simulink model "PassVeh7DOF"  (R2024b)
settings: Solver=ode14x  StartTime=0.0  StopTime=30  FixedStep=0.001  RelTol=1e-1
model workspace (MAT data in the model file):
  A_mu = 10
  B_reff = 8.386
  CONVERTER_DATA = [0 0.1 0.2 0.3 0.4 0.5 0.6 0.7 0.8 0.81 0.82 0.83 ... (63 elements, 21x3)]
  Cps = 2
  Cz = 7766.25
  DOWN_TABLE = [0 0 0 0 0 0 5 5 7.5 7.5 15 15 ... (30 elements, 6x5)]
  DOWN_TH_BP = [0 5 40 50 90 100]
  D_reff = 0.25826
  EMAP = [-40 215 245 264 264 267 267 267 267 267 -44 117 ... (110 elements, 10x11)]
  F0z = [6086.4 4324.8]
  F_reff = 0.07394
  F_zmax = 10000
  F_zmin = 100
  F_zo = 4000
  Kz = 48000
  MF : object (value not decoded)
  NCyl = 6
  NE_VEC = [800 1200 1600 2000 2400 2800 3200 3600 4000 4400 4800]
  Pstd = 101325
  R_eff = 0.298
  Rair = 287
  SUS : object (value not decoded)
  TH_VEC = [0; 20; 30; 40; 50; 60; 70; 80; 90; 100]
  TWAITdn = 1.25
  TWAITup = 0.1
  Tin = [1 2 3 4 5 6 7 8 9 10 2 2 ... (20 elements, 10x2)]
  Tstd = 293.15
  UP_TABLE = [7.5 7.5 15 25 40 40 25 25 35 45 70 80 ... (30 elements, 6x5)]
  UP_TH_BP = [0 25 35 50 90 100]
  VEH : object (value not decoded)
  V_o = 16.7
  V_xlow = 1
  Vd = 0.00346
  WH : object (value not decoded)
  a = 1.515
  alpha_max = 1.5
  alpha_min = -1.5
  b = 1.504
  c_zo = 209651
  epsilon = 0.1
  f_air = [0 0 0 0 0 0 0 0 0 0 0 0 ... (256 elements, 16x16)]
  f_co = [0 0 0 0 0 0 0 0 0 0 0 0 ... (256 elements, 16x16)]
  f_co2 = [0 0 0 0 0 0 0 0 0 0 0 0 ... (256 elements, 16x16)]
  f_eff = [352.135682859 352.135682859 320.724378192 303.655312657 295.930136708 291.240087194 291.240271258 291.240312459 291.240275452 291.240198499 291.240100781 291.240018769 ... (256 elements, 16x16)]
  f_fuel = [0 0 0 0 0 0 0 0 0 0 0 0 ... (256 elements, 16x16)]
  f_hc = [0 0 0 0 0 0 0 0 0 0 0 0 ... (256 elements, 16x16)]
  f_nox = [0 0 0 0 0 0 0 0 0 0 0 0 ... (256 elements, 16x16)]
  f_pm = [0 0 0 0 0 0 0 0 0 0 0 0 ... (256 elements, 16x16)]
  f_susp_axl_bp = [1 2]
  f_susp_dz_bp = [-4 -0.14 -0.13 -0.12 -0.11 -0.1 -0.09 -0.08 -0.07 -0.06 -0.05 -0.04 ... (31 elements, 1x31)]
  f_susp_dzdot_bp = [-4 -0.14 -0.13 -0.12 -0.11 -0.1 -0.09 -0.08 -0.07 -0.06 -0.05 -0.04 ... (31 elements, 1x31)]
  f_susp_fmz = [-213379.591456 -28099.591456 -27619.591456 -27139.591456 -26659.591456 -26179.591456 -25699.591456 -25219.591456 -24739.591456 -24259.591456 -23779.591456 -23299.591456 ... (468968 elements, 31x31x61x2x4)]
  f_susp_geom = [-0.832564012244 0.043269987756 0.045538987756 0.047807987756 0.050076987756 0.052345987756 0.054614987756 0.056883987756 0.059152987756 0.061421987756 0.063690987756 0.065959987756 ... (11346 elements, 31x61x2x3)]
  f_susp_strgdelta_bp = [-0.523598775598 -0.506145483078 -0.488692190558 -0.471238898038 -0.453785605519 -0.436332312999 -0.418879020479 -0.401425727959 -0.383972435439 -0.366519142919 -0.349065850399 -0.331612557879 ... (61 elements, 1x61)]
  f_tbrake = [0 76.8593923996 105.140482948 131.533638111 157.926793274 176.658631717 176.65727296 176.656856686 176.656879077 176.657093756 176.657404516 176.65772406 ... (256 elements, 16x16)]
  f_tbrake_n_bpt = [0 649.519052838 912.419621844 1175.32019085 1438.22075986 1701.12132886 1964.02189787 2226.92246687 2489.82303588 2752.72360489 3015.62417389 3278.5247429 ... (16 elements, 1x16)]
  f_tbrake_t_bpt = [0 34.6410161514 61.0341713143 87.4273264773 113.82048164 140.213636803 166.606791966 192.999947129 219.393102292 245.786257455 272.179412618 298.572567781 ... (16 elements, 1x16)]
  f_texh = [766.752464599 766.752464599 786.17542386 801.679939032 884.591982581 910.574397722 910.571871054 910.570774534 910.570601632 910.570821151 910.571247242 910.571639815 ... (256 elements, 16x16)]
  f_twc_eff_co = [0.17 0.25 0.45 0.99 0.99 0.99 0.99]
  f_twc_eff_hc = [0.21 0.375 0.75 0.98 0.98 0.98 0.98]
  f_twc_eff_lam = [0.909090909 0.944055944 0.979020979 1 1.013986014 1.048951049 1.083916084]
  f_twc_eff_nox = [0.98 0.98 0.98 0.97 0.05 0.02 0]
  h = 0.134
  k_z = 50
  kappa_max = 1.5
  kappa_min = -1.5
  lam_Cx = 1
  lam_Cy = 1
  lam_Cz = 1
  lam_Ex = 1
  lam_Ey = 1
  lam_F_zo = 1
  lam_Hx = 1
  lam_Hy = 1
  lam_Kxkappa = 1
  lam_Kyalpha = 1
  lam_Kygamma = 1
  lam_Kzgamma = 1
  lam_Mr = 1
  lam_Mx = 1
  lam_My = 1
  lam_S = 1
  lam_VMx = 1
  lam_Vx = 1
  lam_Vy = 1
  lam_Vykappa = 1
  lam_muV = 0
  lam_mux = 1
  lam_muy = 1
  lam_t = 1
  lam_xalpha = 1
  lam_ykappa = 1
  numWheel = 4
  p_Cx1 = 1.579
  p_Cy1 = 1.3332
  p_Dx1 = 1.0422
  p_Dx2 = -0.08285
  p_Dx3 = 0
  p_Dy1 = 0.8784
  p_Dy2 = -0.06445
  p_Dy3 = 0
  p_Ex1 = 0.11185
  p_Ex2 = 0.3127
  p_Ex3 = 0
  p_Ex4 = 0.001603
  p_Ey1 = -0.8227
  p_Ey2 = -0.6062
  p_Ey3 = 0.09825
  p_Ey4 = -6.546
  p_Ey5 = 0
  p_Fz1 = 0.7098
  p_Hx1 = 0.00021585
  p_Hx2 = 0.0011538
  p_Hy1 = -0.0018043
  p_Hy2 = 0.003518
  p_Kx1 = 21.69
  p_Kx2 = 13.774
  p_Kx3 = -0.4119
  p_Ky1 = -15.314
  p_Ky2 = 1.7044
  p_Ky3 = 0.36986
  p_Ky4 = 1.9896
  p_Ky5 = 0
  p_Ky6 = -0.9004
  p_Ky7 = -0.2328
  p_Vx1 = 1.5973e-05
  p_Vx2 = 0.0001043
  p_Vy1 = -0.006642
  p_Vy2 = 0.03597
  p_Vy3 = -0.1621
  p_Vy4 = -0.4908
  p_pmx1 = 0
  p_px1 = -0.3489
  p_px2 = 0.382
  p_px3 = -0.09634
  p_px4 = 0.06447
  p_py1 = -0.6249
  p_py2 = -0.06535
  p_py3 = -0.1668
  p_py4 = 0.2834
  p_py5 = 0
  path : object (value not decoded)
  pio = 220000
  q_Fcx = 0
  q_Fz2 = 15.4
  q_Fzy = 0
  q_reo = 0.9974
  q_sx1 = -0.007764
  q_sx10 = 0.2824
  q_sx11 = 5.349
  q_sx12 = 0
  q_sx13 = 0
  q_sx14 = 0
  q_sx2 = 1.1915
  q_sx3 = 0.013948
  q_sx4 = 4.912
  q_sx5 = 1.02
  q_sx6 = 22.83
  q_sx7 = 0.7104
  q_sx8 = -0.023393
  q_sx9 = 0.6581
  q_sy1 = 0.00702
  q_sy2 = 0
  q_sy3 = 0.001515
  q_sy4 = 8.514e-05
  q_sy5 = 0
  q_sy6 = 0
  q_sy7 = 0.9008
  q_sy8 = -0.4089
  q_v1 = 0.0007742
  q_v2 = 0.04667
  r_Bx1 = 12.531
  r_Bx2 = 9.532
  r_Bx3 = 0
  r_By1 = 10.615
  r_By2 = 7.705
  r_By3 = 3.433e-06
  r_By4 = 0
  r_Cx1 = 1.019
  r_Cy1 = 1.0585
  r_Ex1 = -0.4487
  r_Ex2 = -0.4726
  r_Ey1 = 0.3132
  r_Ey2 = 7.63e-06
  r_Hx1 = 0.0002374
  r_Hy1 = 0.011646
  r_Hy2 = 7.63e-06
  r_Vy1 = 0.05654
  r_Vy2 = 7.63e-06
  r_Vy3 = 0
  r_Vy4 = 99.9
  r_Vy5 = 2
  r_Vy6 = 15.814
  r_o = 0.3135
  reqTmaxT = [nan 0.285774810084 0.647179872268 nan nan nan nan nan nan nan nan nan ... (168 elements, 21x8)]
  vehSpd = [0 2.77777777778 5.55555555556 8.33333333333 11.1111111111 13.8888888889 16.6666666667 19.4444444444 22.2222222222 25 27.7777777778 30.5555555556 ... (21 elements, 1x21)]
  vehWidth = 2
  w = 1
symbols that are objects in the model workspace (value not decoded): VEH
undefined symbols (not defined in the file or in its folder): Fzz, Fzzdot, InertFrm, pFz, psi, vdyntiremask, x_o, zdotFz, zFz
libraries: simulink x4, sharedTrackingLibrary x1, mcbcontrolslib x1
(part 12 of 24)

== system PassVeh7DOF/Vehicle Body 3DOF External Longitudinal Wheels/Dual/Vehicle Body 3DOF Dual Track/Signal Routing/Signal Routing/Lateral 3DOF ==
  InertCg : Inport
  BdyFrmCg : Inport  Port=2
  Forces : Inport  Port=3
  Power : Inport  Port=4
  Moments : Inport  Port=5
  WhlAngF : Inport  Port=6  Unit=rad
  WhlAngR : Inport  Port=7  Unit=rad
  Bus Creator1 : BusCreator  Inputs=8
  Bus Creator2 : BusCreator  Inputs=5
  Bus Creator3 : BusCreator  Inputs=2
  Bus Creator4 : BusCreator  Inputs=2
  Bus Selector : BusSelector  OutputSignals=Pwr,PwrInfo
  Demux : Demux  Outputs=2
  Demux1 : Demux  Outputs=2
  Hard Point Coordinate Transform Front : Subsystem  mask(Hard Point Coordinate Transform){R_T1=a, R_T2=0, R_T3=h, aMode=aMode}
      mask prompts: R_T1 "x position from CG to suspension hardpoint:"; R_T2 "y position from CG to suspension hardpoint:"; R_T3 "z position from CG to suspension hardpoint:"
  Hard Point Coordinate Transform Geometric : Subsystem
  Hard Point Coordinate Transform Rear : Subsystem  mask(Hard Point Coordinate Transform){R_T1=-b, R_T2=0, R_T3=h, aMode=aMode}
      mask prompts: R_T1 "x position from CG to suspension hardpoint:"; R_T2 "y position from CG to suspension hardpoint:"; R_T3 "z position from CG to suspension hardpoint:"
  Hitch Coordinate Transform : Subsystem
  InertFrm : Outport  VectorParamsAs1DForOutWhenUnconnected=off
  BdyFrm : Outport  Port=2  VectorParamsAs1DForOutWhenUnconnected=off
  PwrInfo : Outport  Port=3  VectorParamsAs1DForOutWhenUnconnected=off
  wires:
  Hitch Coordinate Transform/1(Inert) -> Bus Creator2/4  "Hitch"
  Hitch Coordinate Transform/2(Body) -> Bus Creator1/6  "Hitch"
  Bus Creator2/1 -> InertFrm/1
  InertCg/1 -> Hard Point Coordinate Transform Geometric/1(InertFrmCg), Hitch Coordinate Transform/1(InertFrmCg), Hard Point Coordinate Transform Rear/1(InertFrmCg), Hard Point Coordinate Transform Front/1(InertFrmCg), Bus Creator2/1  "Cg"
  Hard Point Coordinate Transform Front/1(Inertial) -> Bus Creator2/2  "FrntAxl"
  Hard Point Coordinate Transform Rear/2(Body) -> Bus Creator1/5  "RearAxl"
  Bus Creator1/1 -> BdyFrm/1  "BdyFrm"
  Hard Point Coordinate Transform Rear/1(Inertial) -> Bus Creator2/3  "RearAxl"
  Hard Point Coordinate Transform Front/2(Body) -> Bus Creator1/4  "FrntAxl"
  Forces/1 -> Bus Creator1/2  "Forces"
  Bus Selector/1 -> Bus Creator1/7  "<Pwr>"
  Moments/1 -> Bus Creator1/3  "Moments"
  BdyFrmCg/1 -> Hard Point Coordinate Transform Front/2(BdyFrmCg), Hitch Coordinate Transform/2(BodyFrmCg), Bus Creator1/1, Hard Point Coordinate Transform Geometric/2(BdyFrmCg), Hard Point Coordinate Transform Rear/2(BdyFrmCg)  "Cg"
  Hard Point Coordinate Transform Geometric/1(Inert) -> Bus Creator2/5  "Geom"
  Hard Point Coordinate Transform Geometric/2(Body) -> Bus Creator1/8  "Geom"
  Bus Creator3/1 -> Hard Point Coordinate Transform Front/3(Steer)  "Steer"
  WhlAngF/1 -> Demux/1  "WhlAngF"
  WhlAngR/1 -> Demux1/1  "WhlAngR"
  Bus Creator4/1 -> Hard Point Coordinate Transform Rear/3(Steer)  "Steer"
  Demux/2 -> Bus Creator3/2  "WhlAngFR"
  Demux1/1 -> Bus Creator4/1  "WhlAngRL"
  Demux1/2 -> Bus Creator4/2  "WhlAngRR"
  Demux/1 -> Bus Creator3/1  "WhlAngFL"
  Bus Selector/2 -> PwrInfo/1  "<PwrInfo>"
  Power/1 -> Bus Selector/1  "Pwr"

== system PassVeh7DOF/Vehicle Body 3DOF External Longitudinal Wheels/Dual/Vehicle Body 3DOF Dual Track/Signal Routing/Signal Routing/Moments ==
  MBody : Inport
  Mdrag : Inport  Port=2
  MExt : Inport  Port=3
  Mh : Inport  Port=4
  Bus Creator{1..3,24} (4 alike) : BusCreator  Inputs=3
  Bus Creator7 : BusCreator  Inputs=4
  Demux{,1..3} (4 alike) : Demux  Outputs=3
  Signal Specification{1..11,23} (12 alike) : SignalSpecification  Unit=N*m
  Moments : Outport  VectorParamsAs1DForOutWhenUnconnected=off
  wires:
  Signal Specification10/1 -> Bus Creator2/3  "Mz"
  Demux3/3 -> Signal Specification10/1
  Demux3/1 -> Signal Specification11/1
  Signal Specification11/1 -> Bus Creator2/1  "Mx"
  Mh/1 -> Demux3/1
  Demux3/2 -> Signal Specification9/1
  Signal Specification9/1 -> Bus Creator2/2  "My"
  Bus Creator2/1 -> Bus Creator7/4  "Hitch"
  Signal Specification23/1 -> Bus Creator24/1  "Mx"
  Bus Creator24/1 -> Bus Creator7/1  "Body"
  Signal Specification1/1 -> Bus Creator24/2  "My"
  Signal Specification2/1 -> Bus Creator24/3  "Mz"
  Bus Creator1/1 -> Bus Creator7/2  "Drag"
  Bus Creator7/1 -> Moments/1  "Moments"
  Demux/2 -> Signal Specification1/1
  Demux/1 -> Signal Specification23/1
  Demux/3 -> Signal Specification2/1
  MBody/1 -> Demux/1
  Mdrag/1 -> Demux1/1
  Demux1/3 -> Signal Specification4/1
  Demux1/1 -> Signal Specification5/1
  Demux1/2 -> Signal Specification3/1
  Signal Specification4/1 -> Bus Creator1/3  "Mz"
  Signal Specification3/1 -> Bus Creator1/2  "My"
  Signal Specification5/1 -> Bus Creator1/1  "Mx"
  MExt/1 -> Demux2/1
  Signal Specification7/1 -> Bus Creator3/3  "Mz"
  Signal Specification6/1 -> Bus Creator3/2  "My"
  Bus Creator3/1 -> Bus Creator7/3  "Ext"
  Signal Specification8/1 -> Bus Creator3/1  "Mx"
  Demux2/2 -> Signal Specification6/1
  Demux2/1 -> Signal Specification8/1
  Demux2/3 -> Signal Specification7/1

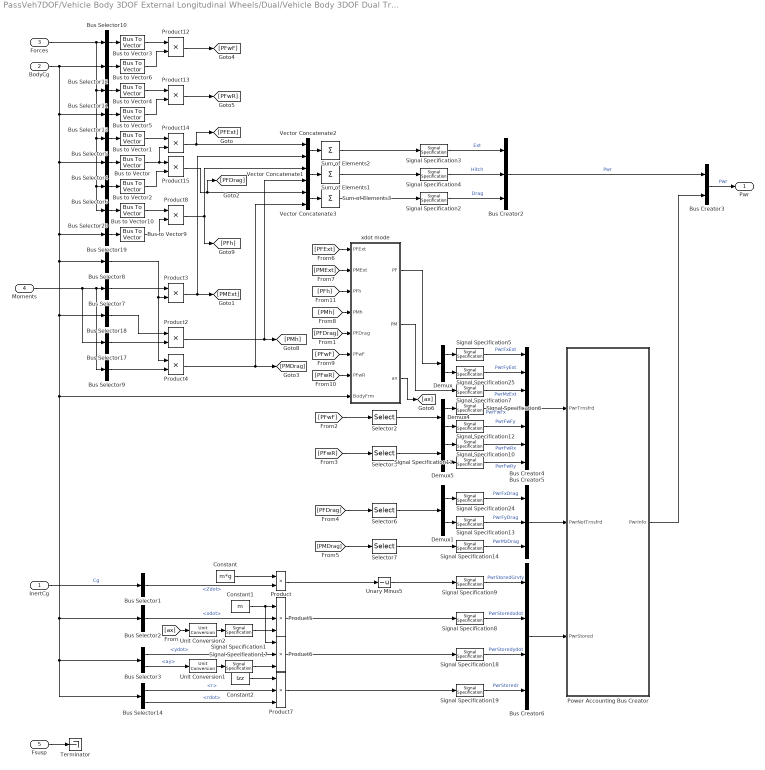
== system PassVeh7DOF/Vehicle Body 3DOF External Longitudinal Wheels/Dual/Vehicle Body 3DOF Dual Track/Signal Routing/Signal Routing/Power ==
  InertCg : Inport
  BodyCg : Inport  Port=2
  Forces : Inport  Port=3
  Moments : Inport  Port=4
  Fsusp : Inport  Port=5
  Bus Creator2 : BusCreator  Inputs=3
  Bus Creator3 : BusCreator  Inputs=2
  Bus Creator4 : BusCreator  Inputs=7
  Bus Creator5 : BusCreator  Inputs=3
  Bus Creator6 : BusCreator  Inputs=4
  Bus Selector1 : BusSelector  OutputSignals=Cg.Vel.Zdot
  Bus Selector10 : BusSelector  OutputSignals=FrntAxl.Fx,FrntAxl.Fy,FrntAxl.Fz  OutputAsBus=on
  Bus Selector11 : BusSelector  OutputSignals=RearAxl.Fx,RearAxl.Fy,RearAxl.Fz  OutputAsBus=on
  Bus Selector12 : BusSelector  OutputSignals=FrntAxl.Vel.xdot,FrntAxl.Vel.ydot,FrntAxl.Vel.zdot  OutputAsBus=on
  Bus Selector13 : BusSelector  OutputSignals=RearAxl.Vel.xdot,RearAxl.Vel.ydot,RearAxl.Vel.zdot  OutputAsBus=on
  Bus Selector14 : BusSelector  OutputSignals=Cg.AngVel.r,Cg.AngAcc.rdot
  Bus Selector17 : BusSelector  OutputSignals=Hitch.Mx,Hitch.My,Hitch.Mz  OutputAsBus=on
  Bus Selector18 : BusSelector  OutputSignals=Cg.AngVel.p,Cg.AngVel.q,Cg.AngVel.r  OutputAsBus=on
  Bus Selector19 : BusSelector  OutputSignals=Hitch.Vel.xdot,Hitch.Vel.ydot,Hitch.Vel.zdot  OutputAsBus=on
  Bus Selector2 : BusSelector  OutputSignals=Cg.Vel.xdot
  Bus Selector20 : BusSelector  OutputSignals=Hitch.Fx,Hitch.Fy,Hitch.Fz  OutputAsBus=on
  Bus Selector3 : BusSelector  OutputSignals=Cg.Vel.ydot,Cg.Acc.ay
  Bus Selector4 : BusSelector  OutputSignals=Cg.Vel.xdot,Cg.Vel.ydot,Cg.Vel.zdot  OutputAsBus=on
  Bus Selector5 : BusSelector  OutputSignals=Ext.Fx,Ext.Fy,Ext.Fz  OutputAsBus=on
  Bus Selector6 : BusSelector  OutputSignals=Drag.Fx,Drag.Fy,Drag.Fz  OutputAsBus=on
  Bus Selector7 : BusSelector  OutputSignals=Ext.Mx,Ext.My,Ext.Mz  OutputAsBus=on
  Bus Selector8 : BusSelector  OutputSignals=Cg.AngVel.p,Cg.AngVel.q,Cg.AngVel.r  OutputAsBus=on
  Bus Selector9 : BusSelector  OutputSignals=Drag.Mx,Drag.My,Drag.Mz  OutputAsBus=on
  Bus to Vector{,1..6,9..10} (9 alike) : BusToVector
  Constant : Constant  Value=m*g
  Constant1 : Constant  Value=m
  Constant2 : Constant  Value=Izz
  Demux{,1,4..5} (4 alike) : Demux  Outputs=2
  Power Accounting Bus Creator : Subsystem  mask(Power Accounting Bus Creator){AssctBlkSelPopup=Parent reference block, RefBlkName='autolibshared/Vehicle Body 3DOF Single Track', PwrTrnsfrdCheckBox=on, PwrNotTrnsfrdCheckBox=on, PwrStoredCheckBox=on, aMode=aMode}
      mask prompts: AssctBlkSelPopup "autoblks_shared:autoblkPwrInfoBus:assocBlkSel"; RefBlkName "autoblks_shared:autoblkPwrInfoBus:refBlkName"
      mask init:
      | autosharedicon('autolibpowerbusutil', gcb, 'Initialization')
      settings: ModelCloseFcn=autosharedicon('autolibpowerbusutil', gcb, 'CloseFcn')  OpenFcn=autosharedicon('autolibpowerbusutil', gcb, 'OpenFcn')  CloseFcn=autosharedicon('autolibpowerbusutil', gcb, 'CloseFcn')
      mask Help: eval('autosharedhelp(''pbpwrbuscreator'')');
      mask TypeOptions AssctBlkSelPopup: Parent | Parent reference block
      mask DialogControl AssctBlkSelPopup Prompt: Associated block selection:
      mask DialogControl RefBlkName Prompt: Reference block name:
  Product{,2..4,8,12..15} (9 alike) : Product
  Product5 : Product  Inputs=3
  Product6 : Product  Inputs=3
  Product7 : Product  Inputs=3
  Selector2 : Selector  InputPortWidth=3  IndexOptions=Index vector (dialog)  Indices=[1 2]  OutputSizes=1
  Selector3 : Selector  InputPortWidth=3  IndexOptions=Index vector (dialog)  Indices=[1 2]  OutputSizes=1
  Selector6 : Selector  InputPortWidth=3  IndexOptions=Index vector (dialog)  Indices=[1 2]  OutputSizes=1
  Selector7 : Selector  InputPortWidth=3  IndexOptions=Index vector (dialog)  Indices=[3]  OutputSizes=1
  Signal Specification1 : SignalSpecification  Unit=m/s^2
  Signal Specification{2..14,18..19,24..25} (17 alike) : SignalSpecification  Unit=W
  Signal Specification17 : SignalSpecification  Unit=m/s^2
  Sum of Elements1 : Sum  Inputs=+
  Sum of Elements2 : Sum  Inputs=+
  Sum of Elements3 : Sum  Inputs=+
  Terminator : Terminator
  Unary Minus5 : UnaryMinus
  Unit Conversion1 : UnitConversion
  Unit Conversion2 : UnitConversion
  Vector Concatenate1 : Concatenate
  Vector Concatenate2 : Concatenate
  Vector Concatenate3 : Concatenate
  xdot mode : Subsystem  Variant=on  VariantControlMode=label  LabelModeActiveChoice=1
  Pwr : Outport  VectorParamsAs1DForOutWhenUnconnected=off
  wires:
  [PMh] -> xdot mode/4(PMh)
  [PFh] -> xdot mode/3(PFh)
  Vector Concatenate1/1 -> Sum of Elements1/1
  Sum of Elements1/1 -> Signal Specification4/1
  Signal Specification4/1 -> Bus Creator2/2  "Hitch"
  Bus Selector19/1 -> Bus to Vector9/1
  Bus to Vector9/1 -> Product8/2
  Bus to Vector10/1 -> Product8/1
  Bus Selector20/1 -> Bus to Vector10/1
  Product8/1 -> [PFh], Vector Concatenate1/1
  Product2/1 -> Vector Concatenate1/2, [PMh]
  BodyCg/1 -> Bus Selector4/1, Bus Selector8/1, Bus Selector18/1, xdot mode/8(BodyFrm), Bus Selector2/1, Bus Selector14/1, Bus Selector3/1, Bus Selector19/1, Bus Selector13/1, Bus Selector12/1
  Moments/1 -> Bus Selector7/1, Bus Selector9/1, Bus Selector17/1
  Bus Selector18/1 -> Product2/1
  Bus Selector17/1 -> Product2/2
  Signal Specification3/1 -> Bus Creator2/1  "Ext"
  Product15/1 -> Vector Concatenate3/1, [PFDrag]
  Bus Creator2/1 -> Bus Creator3/1  "Pwr"
  Product14/1 -> [PFExt], Vector Concatenate2/1
  Bus Selector5/1 -> Bus to Vector1/1
  Bus Selector1/1 -> Product/2  "<Zdot>"
  Product3/1 -> [PMExt], Vector Concatenate2/2
  Bus Selector11/1 -> Bus to Vector4/1
  InertCg/1 -> Bus Selector1/1  "Cg"
  Sum of Elements3/1 -> Signal Specification2/1
  Bus to Vector1/1 -> Product14/1
  Bus Selector6/1 -> Bus to Vector2/1
  Signal Specification8/1 -> Bus Creator6/2  "PwrStoredxdot"
  [PFwR] -> Selector3/1
  Demux/2 -> Signal Specification25/1
  Product13/1 -> [PFwR]
  Product7/1 -> Signal Specification19/1
  Bus Selector3/1 -> Product6/2  "<ydot>"
  Constant2/1 -> Product7/1
  Sum of Elements2/1 -> Signal Specification3/1
  Bus to Vector2/1 -> Product15/2
  Bus Selector13/1 -> Bus to Vector5/1
  Vector Concatenate2/1 -> Sum of Elements2/1
  Signal Specification19/1 -> Bus Creator6/4  "PwrStoredr"
  Bus Selector2/1 -> Product5/2  "<xdot>"
  Vector Concatenate3/1 -> Sum of Elements3/1
  Signal Specification18/1 -> Bus Creator6/3  "PwrStoredydot"
  Bus Selector14/2 -> Product7/3  "<rdot>"
  Bus Selector14/1 -> Product7/2  "<r>"
  Forces/1 -> Bus Selector6/1, Bus Selector20/1, Bus Selector5/1, Bus Selector11/1, Bus Selector10/1
  xdot mode/1(PF) -> Demux/1
  Bus Selector10/1 -> Bus to Vector3/1
  Bus to Vector6/1 -> Product12/2
  [PMDrag] -> Selector7/1
  Signal Specification14/1 -> Bus Creator5/3  "PwrMzDrag"
  [PFwF] -> Selector2/1
  Signal Specification7/1 -> Bus Creator4/3  "PwrMzExt"
  Bus Selector4/1 -> Bus to Vector/1
  Bus to Vector3/1 -> Product12/1
  Signal Specification13/1 -> Bus Creator5/2  "PwrFyDrag"
  [PFDrag] -> Selector6/1
  Selector6/1 -> Demux1/1
  Bus Selector12/1 -> Bus to Vector6/1
  Signal Specification6/1 -> Bus Creator4/4  "PwrFwFx"
  Bus Creator3/1 -> Pwr/1  "Pwr"
  Bus to Vector4/1 -> Product13/1
  Signal Specification9/1 -> Bus Creator6/1  "PwrStoredGrvty"
  Signal Specification11/1 -> Bus Creator4/7  "PwrFwRy"
  xdot mode/2(PM) -> Signal Specification7/1
  Bus Selector7/1 -> Product3/1
  Signal Specification2/1 -> Bus Creator2/3  "Drag"
  Bus Selector8/1 -> Product3/2, Product4/1
  Signal Specification10/1 -> Bus Creator4/6  "PwrFwRx"
  Signal Specification12/1 -> Bus Creator4/5  "PwrFwFy"
  Selector2/1 -> Demux4/1
  Demux5/2 -> Signal Specification11/1
  Bus Selector9/1 -> Product4/2
  Selector3/1 -> Demux5/1
  Demux4/1 -> Signal Specification6/1
  Demux1/1 -> Signal Specification24/1
  Product12/1 -> [PFwF]
  Unary Minus5/1 -> Signal Specification9/1
  Signal Specification24/1 -> Bus Creator5/1  "PwrFxDrag"
  Demux5/1 -> Signal Specification10/1
  Signal Specification5/1 -> Bus Creator4/1  "PwrFxExt"
  Bus Creator6/1 -> Power Accounting Bus Creator/3(PwrStored)
  Bus to Vector/1 -> Product15/1, Product14/2
  Constant1/1 -> Product6/1, Product5/1
  Signal Specification25/1 -> Bus Creator4/2  "PwrFyExt"
  Product/1 -> Unary Minus5/1
  Bus Creator5/1 -> Power Accounting Bus Creator/2(PwrNotTrnsfrd)
  Bus to Vector5/1 -> Product13/2
  Bus Creator4/1 -> Power Accounting Bus Creator/1(PwrTrnsfrd)
  Demux/1 -> Signal Specification5/1
  Product6/1 -> Signal Specification18/1
  Constant/1 -> Product/1
  Demux4/2 -> Signal Specification12/1
  Power Accounting Bus Creator/1(PwrInfo) -> Bus Creator3/2
  Product4/1 -> [PMDrag], Vector Concatenate3/2
  Fsusp/1 -> Terminator/1
  [PFExt] -> xdot mode/1(PFExt)
  [PMExt] -> xdot mode/2(PMExt)
  [PFDrag] -> xdot mode/5(PFDrag)
  [PFwF] -> xdot mode/6(PFwF)
  [PFwR] -> xdot mode/7(PFwR)
  Product5/1 -> Signal Specification8/1
  Signal Specification17/1 -> Product6/3
  Unit Conversion1/1 -> Signal Specification17/1
  Bus Selector3/2 -> Unit Conversion1/1  "<ay>"
  Selector7/1 -> Signal Specification14/1
  Demux1/2 -> Signal Specification13/1
  Signal Specification1/1 -> Product5/3
  Unit Conversion2/1 -> Signal Specification1/1
  xdot mode/3(ax) -> [ax]
  [ax] -> Unit Conversion2/1

== system PassVeh7DOF/Vehicle Body 3DOF External Longitudinal Wheels/Dual/Vehicle Body 3DOF Dual Track/Signal Routing/Signal Routing/state2bus ==
  x : Inport
  y : Inport  Port=2
  Xo : Inport  Port=3
  Angle Wrap : Subsystem  Variant=on  VariantControlMode=label  VariantControl=Variant1  LabelModeActiveChoice=Wrap
  Body Slip : Subsystem
  Bus Creator1 : BusCreator  Inputs=6
  Bus Creator{3,6..7,10..11,13..14} (7 alike) : BusCreator  Inputs=3
  Bus Creator15 : BusCreator  Inputs=6
  Bus Creator2 : BusCreator  Inputs=1
  COMB2I : MATLAB Function  TreatAsAtomicUnit=on
  Constant{,1..10} (11 alike) : Constant  Value=0
  Demux{1..2,4,6} (4 alike) : Demux  Outputs=2
  Demux3 : Demux  Outputs=3
  Demux5 : Demux  Outputs=3
  Integrator : Integrator  InitialConditionSource=external
  Rotation Angles to Direction Cosine Matrix : Subsystem  mask(Ang2DCM){rotationOrder=ZYX, aMode=aMode}
      mask prompts: rotationOrder "shared_aeroblks:sharedaeroblktransform:blockAng2DCMParamRotationOrder"
      mask help: shared_aeroblks:sharedaeroblktransform:blockAng2DCMDesc
      mask init:
      | if aerosharedtest(gcb)
      |     ports=aerosharedicon('sharedang2dcm');
      | else
      |     ports=sharedautoicon('sharedang2dcm');
      | end
      settings: AttributesFormatString=Rotation Order: %<rotationOrder>
      mask Help: eval('if license(''test'',''Aerospace_Blockset'')aerosharedhelp(''rotation_angles_to_direction_cosine_matrix'');elseif license(''test'',''Powertrain_Blockset'')sharedautohelp(''rotation_angles_to_direction_cosine_matrix'');end')
      mask TypeOptions rotationOrder: shared_aeroblks:sharedaeroblktransform:blockParamComboZYX | shared_aeroblks:sharedaeroblktransform:blockParamComboZYZ | shared_aeroblks:sharedaeroblktransform:blockParamComboZXY | shared_aeroblks:sharedaeroblktransform:blockParamComboZXZ | shared_aeroblks:sharedaeroblktransform:blockParamComboYXZ | shared_aeroblks:sharedaeroblktransform:blockParamComboYXY | shared_aeroblks:sharedaeroblktransform:blockParamComboYZX | shared_aeroblks:sharedaeroblktransform:blockParamComboYZY | shared_aeroblks:sharedaeroblktransform:blockParamComboXYZ | shared_aeroblks:sharedaeroblktransform:blockParamComboXYX | shared_aeroblks:sharedaeroblktransform:blockParamComboXZY | shared_aeroblks:sharedaeroblktransform:blockParamComboXZX
      mask DialogControl rotationOrder Prompt: Rotation order:
      mask Display:
      | port_label('input',1,'[R_1,R_2,R_3]','texmode','on')
      | port_label('output',1,'DCM_{be}','texmode','on')
  Selector : Selector  InputPortWidth=3  IndexOptions=Index vector (dialog)  Indices=[3 2 1]  OutputSizes=1
  Selector1 : Selector  IndexOptions=Index vector (dialog)  Indices=[3]  OutputSizes=1
  Selector2 : Selector  IndexOptions=Index vector (dialog)  Indices=[3,1,2]  OutputSizes=1
  Selector3 : Selector  IndexOptions=Index vector (dialog)  Indices=[1,2]  OutputSizes=1
  Selector4 : Selector  IndexOptions=Index vector (dialog)  Indices=[4,1,2]  OutputSizes=1
  Signal Specification : SignalSpecification  Unit=gn
  Signal Specification1 : SignalSpecification  Unit=rad/s
  Signal Specification{4..6,10..12} (6 alike) : SignalSpecification  Unit=m/s
  Signal Specification13 : SignalSpecification  Unit=m
  Signal Specification14 : SignalSpecification  Unit=m
  Signal Specification15 : SignalSpecification  Unit=m
  Signal Specification16 : SignalSpecification  Unit=m/s^2
  Signal Specification17 : SignalSpecification  Unit=m/s^2
  Signal Specification18 : SignalSpecification  Unit=m/s^2
  Signal Specification19 : SignalSpecification  Unit=rad/s^2
  Signal Specification2 : SignalSpecification  Unit=rad/s
  Signal Specification20 : SignalSpecification  Unit=rad/s^2
  Signal Specification21 : SignalSpecification  Unit=rad/s^2
  Signal Specification3 : SignalSpecification  Unit=rad/s
  Signal Specification7 : SignalSpecification  Unit=rad
  Signal Specification8 : SignalSpecification  Unit=rad
  Signal Specification9 : SignalSpecification  Unit=rad
  xddot2ax : Subsystem
  COM_I : Outport  VectorParamsAs1DForOutWhenUnconnected=off
  COM_B : Outport  Port=2  VectorParamsAs1DForOutWhenUnconnected=off
  wires:
  [angles] -> Selector/1
  Selector/1 -> Rotation Angles to Direction Cosine Matrix/1(In1)
  Rotation Angles to Direction Cosine Matrix/1(Out1) -> Bus Creator15/6  "DCM"
  Angle Wrap/1(" y") -> Signal Specification7/1
  Selector1/1 -> Signal Specification21/1
  Constant10/1 -> Signal Specification20/1
  Constant9/1 -> Signal Specification19/1
  Bus Creator3/1 -> Bus Creator15/5  "AngAcc"
  Signal Specification20/1 -> Bus Creator3/1  "pdot"
  Signal Specification19/1 -> Bus Creator3/2  "qdot"
  Signal Specification21/1 -> Bus Creator3/3  "rdot"
  Xo/1 -> Integrator/2
  Body Slip/1(Beta) -> Bus Creator2/1  "Beta"
  Bus Creator2/1 -> Bus Creator15/2  "Ang"
  Bus Creator1/1 -> Bus Creator15/4  "Acc"
  Constant8/1 -> Signal Specification10/1
  Demux6/2 -> Signal Specification17/1
  Demux6/1 -> Signal Specification16/1
  Constant1/1 -> Signal Specification/1  "az"
  Signal Specification16/1 -> Bus Creator1/4  "xddot"
  Signal Specification17/1 -> Bus Creator1/5  "yddot"
  Signal Specification18/1 -> Bus Creator1/6  "zddot"
  Constant3/1 -> Signal Specification18/1  "zddot"
  Selector3/1 -> Demux6/1, Demux4/1
  y/1 -> Selector3/1, Selector1/1
  Signal Specification/1 -> Bus Creator1/3  "az"
  Signal Specification7/1 -> Bus Creator11/3  "psi"
  COMB2I/1(y) -> Demux1/1, Integrator/1
  Integrator/1 -> Demux2/1
  Signal Specification6/1 -> Bus Creator14/2  "ydot"
  Bus Creator11/1 -> Bus Creator7/3, [angles]  "Ang"
  Signal Specification5/1 -> Bus Creator14/1  "xdot"
  Bus Creator15/1 -> COM_B/1  "COM_B"
  Signal Specification2/1 -> Bus Creator13/2  "q"
  Signal Specification12/1 -> Bus Creator6/2  "Ydot"
  Selector2/1 -> Demux3/1
  Signal Specification8/1 -> Bus Creator11/2  "theta"
  Bus Creator10/1 -> Bus Creator7/1  "Disp"
  Bus Creator6/1 -> Bus Creator7/2  "Vel"
  Bus Creator14/1 -> Bus Creator15/1  "Vel"
  Signal Specification3/1 -> Bus Creator13/1  "p"
  Bus Creator7/1 -> COM_I/1  "COM_I"
  Signal Specification9/1 -> Bus Creator11/1  "phi"
  Signal Specification14/1 -> Bus Creator10/1  "X"
  Signal Specification13/1 -> Bus Creator10/3  "Z"
  Bus Creator13/1 -> Bus Creator15/3  "AngVel"
  Signal Specification15/1 -> Bus Creator10/2  "Y"
  Signal Specification11/1 -> Bus Creator6/1  "Xdot"
  Signal Specification4/1 -> Bus Creator14/3  "zdot"
  Signal Specification10/1 -> Bus Creator6/3  "Zdot"
  x/1 -> COMB2I/1(x), Selector2/1, Body Slip/1(x), Selector4/1
  Demux5/1 -> Signal Specification1/1, xddot2ax/1(r)  "r"
  Selector4/1 -> Demux5/1
  Demux5/2 -> xddot2ax/2(xdot)  "xdot"
  Demux5/3 -> xddot2ax/3(ydot)  "ydot"
  Demux4/1 -> xddot2ax/4(xddot)  "xddot"
  Demux4/2 -> xddot2ax/5(yddot)  "yddot"
  xddot2ax/1(ax) -> Bus Creator1/1  "ax"
  xddot2ax/2(ay) -> Bus Creator1/2  "ay"
  Signal Specification1/1 -> Bus Creator13/3  "r"
  Constant5/1 -> Signal Specification2/1
  Constant4/1 -> Signal Specification3/1
  Constant6/1 -> Signal Specification4/1
  Demux3/2 -> Signal Specification5/1
  Demux3/3 -> Signal Specification6/1
  Demux3/1 -> Angle Wrap/1("u ")
  Constant7/1 -> Signal Specification8/1
  Constant2/1 -> Signal Specification9/1
  Demux1/2 -> Signal Specification12/1
  Demux1/1 -> Signal Specification11/1
  Constant/1 -> Signal Specification13/1
  Demux2/2 -> Signal Specification15/1
  Demux2/1 -> Signal Specification14/1

== system PassVeh7DOF/Vehicle Body 3DOF External Longitudinal Wheels/Dual/Vehicle Body 3DOF Dual Track/Signal Routing/Signal Routing Dual/Forces 3DOF ==
  FBody : Inport
  Fdrag : Inport  Port=2
  Fg : Inport  Port=3
  Fs : Inport  Port=4  Unit=N
  Fext : Inport  Port=5
  FTire : Inport  Port=6
  Fh : Inport  Port=7
  Bus Creator{1,3..5,8..9,12..14,17..18,22..23} (13 alike) : BusCreator  Inputs=3
  Bus Creator{2,6..7,10..11} (5 alike) : BusCreator  Inputs=2
  Bus Creator20 : BusCreator  Inputs=8
  Demux{1..5,7..11,13..15} (13 alike) : Demux  Outputs=3
  Demux12 : Demux  Outputs=[3,3,3,3]
  Demux6 : Demux  Outputs=[3,3,3,3]
  Selector : Selector  InputPortWidth=12  IndexOptions=Index vector (dialog)  Indices=[3,6]  OutputSizes=1
  Selector1 : Selector  InputPortWidth=12  IndexOptions=Index vector (dialog)  Indices=[9,12]  OutputSizes=1
  Signal Specification{2..9,14..22} (17 alike) : SignalSpecification  Unit=N
  Forces : Outport  VectorParamsAs1DForOutWhenUnconnected=off
  FzF : Outport  Port=2  VectorParamsAs1DForOutWhenUnconnected=off
  FzR : Outport  Port=3  VectorParamsAs1DForOutWhenUnconnected=off
  wires:
  Demux15/2 -> Signal Specification8/1
  Demux15/1 -> Signal Specification7/1
  Signal Specification9/1 -> Bus Creator14/3  "Fz"
  Signal Specification8/1 -> Bus Creator14/2  "Fy"
  Fh/1 -> Demux15/1
  Demux15/3 -> Signal Specification9/1
  Bus Creator14/1 -> Bus Creator20/3  "Hitch"
  Signal Specification7/1 -> Bus Creator14/1  "Fx"
  Selector1/1 -> FzR/1
  Selector/1 -> FzF/1
  Demux13/3 -> Bus Creator12/3  "Fz"
  Bus Creator13/1 -> Bus Creator11/2  "Rght"
  Demux14/1 -> Bus Creator13/1  "Fx"
  Demux14/2 -> Bus Creator13/2  "Fy"
  Demux14/3 -> Bus Creator13/3  "Fz"
  Demux6/4 -> Demux14/1
  Demux6/3 -> Demux13/1
  Demux13/2 -> Bus Creator12/2  "Fy"
  Demux13/1 -> Bus Creator12/1  "Fx"
  Signal Specification2/1 -> Demux12/1
  Bus Creator12/1 -> Bus Creator11/1  "Lft"
  Bus Creator3/1 -> Bus Creator10/2  "Rght"
  Bus Creator4/1 -> Bus Creator10/1  "Lft"
  Demux12/3 -> Demux10/1
  Demux12/4 -> Demux11/1
  Demux11/1 -> Bus Creator8/1  "Fx"
  Demux11/2 -> Bus Creator8/2  "Fy"
  Demux11/3 -> Bus Creator8/3  "Fz"
  Demux10/3 -> Bus Creator9/3  "Fz"
  Demux10/2 -> Bus Creator9/2  "Fy"
  Demux10/1 -> Bus Creator9/1  "Fx"
  Bus Creator9/1 -> Bus Creator7/1  "Lft"
  Bus Creator8/1 -> Bus Creator7/2  "Rght"
  Bus Creator1/1 -> Bus Creator6/2  "Rght"
  Bus Creator18/1 -> Bus Creator6/1  "Lft"
  Demux1/1 -> Signal Specification14/1
  Fg/1 -> Demux1/1
  Demux1/3 -> Signal Specification16/1
  Demux1/2 -> Signal Specification15/1
  Bus Creator23/1 -> Bus Creator20/8  "Grvty"
  Bus Creator20/1 -> Forces/1  "Forces"
  Signal Specification16/1 -> Bus Creator23/3  "Fz"
  Signal Specification19/1 -> Bus Creator17/3  "Fz"
  Signal Specification14/1 -> Bus Creator23/1  "Fx"
  Signal Specification17/1 -> Bus Creator17/1  "Fx"
  Signal Specification18/1 -> Bus Creator17/2  "Fy"
  Signal Specification21/1 -> Bus Creator22/2  "Fy"
  Signal Specification15/1 -> Bus Creator23/2  "Fy"
  Signal Specification20/1 -> Bus Creator22/1  "Fx"
  Signal Specification22/1 -> Bus Creator22/3  "Fz"
  Bus Creator22/1 -> Bus Creator20/2  "Ext"
  Fext/1 -> Demux3/1
  Demux3/1 -> Signal Specification20/1
  Demux3/2 -> Signal Specification21/1
  Demux3/3 -> Signal Specification22/1
  Demux4/1 -> Signal Specification17/1
  Demux4/2 -> Signal Specification18/1
  Demux4/3 -> Signal Specification19/1
  Fdrag/1 -> Demux4/1
  Bus Creator6/1 -> Bus Creator20/4  "FrntAxl"
  Bus Creator7/1 -> Bus Creator20/5  "RearAxl"
  Demux2/1 -> Bus Creator18/1  "Fx"
  Demux2/2 -> Bus Creator18/2  "Fy"
  Demux2/3 -> Bus Creator18/3  "Fz"
  Demux5/3 -> Bus Creator1/3  "Fz"
  Demux5/2 -> Bus Creator1/2  "Fy"
  Demux8/1 -> Bus Creator3/1  "Fx"
  Demux8/2 -> Bus Creator3/2  "Fy"
  Demux8/3 -> Bus Creator3/3  "Fz"
  Demux7/3 -> Bus Creator4/3  "Fz"
  Demux7/2 -> Bus Creator4/2  "Fy"
  Demux7/1 -> Bus Creator4/1  "Fx"
  Bus Creator11/1 -> Bus Creator2/2  "RearTires"
  Bus Creator10/1 -> Bus Creator2/1  "FrntTires"
  Demux5/1 -> Bus Creator1/1  "Fx"
  Fs/1 -> Signal Specification2/1
  Demux12/2 -> Demux5/1
  Demux12/1 -> Demux2/1
  FTire/1 -> Signal Specification3/1
  Signal Specification3/1 -> Demux6/1, Selector/1, Selector1/1
  Demux6/1 -> Demux7/1
  Demux6/2 -> Demux8/1
  Bus Creator2/1 -> Bus Creator20/6  "Tires"
  Bus Creator17/1 -> Bus Creator20/7  "Drag"
  Bus Creator5/1 -> Bus Creator20/1  "Body"
  Demux9/3 -> Signal Specification6/1
  Demux9/2 -> Signal Specification5/1
  Demux9/1 -> Signal Specification4/1
  FBody/1 -> Demux9/1
  Signal Specification6/1 -> Bus Creator5/3  "Fz"
  Signal Specification4/1 -> Bus Creator5/1  "Fx"
  Signal Specification5/1 -> Bus Creator5/2  "Fy"

== system PassVeh7DOF/Vehicle Body 3DOF External Longitudinal Wheels/Dual/Vehicle Body 3DOF Dual Track/Signal Routing/Signal Routing Dual/Lateral 3DOF ==
  InertCg : Inport
  BdyFrmCg : Inport  Port=2
  Forces : Inport  Port=3
  Power : Inport  Port=4
  Moments : Inport  Port=5
  WhlAngF : Inport  Port=6
  WhlAngR : Inport  Port=7
  Bus Creator1 : BusCreator  Inputs=8
  Bus Creator2 : BusCreator  Inputs=5
  Bus Creator{3..4,7..8} (4 alike) : BusCreator  Inputs=2
  Bus Creator5 : BusCreator  Inputs=3
  Bus Creator6 : BusCreator  Inputs=3
  Bus Selector : BusSelector  OutputSignals=Pwr,PwrInfo
  Demux : Demux  Outputs=2
  Demux1 : Demux  Outputs=2
  Hard Point Coordinate Transform Front Left : Subsystem
  Hard Point Coordinate Transform Front Right : Subsystem
  Hard Point Coordinate Transform Geometric : Subsystem
  Hard Point Coordinate Transform Rear Left : Subsystem
  Hard Point Coordinate Transform Rear Right : Subsystem
  Hitch Coordinate Transform : Subsystem
  InertFrm : Outport  VectorParamsAs1DForOutWhenUnconnected=off
  BdyFrm : Outport  Port=2  VectorParamsAs1DForOutWhenUnconnected=off
  PwrInfo : Outport  Port=3  VectorParamsAs1DForOutWhenUnconnected=off
  wires:
  Hitch Coordinate Transform/2(Body) -> Bus Creator1/6  "Hitch"
  Hitch Coordinate Transform/1(Inert) -> Bus Creator2/4  "Hitch"
  Power/1 -> Bus Selector/1  "Pwr"
  Bus Selector/1 -> Bus Creator1/7  "<Pwr>"
  Bus Selector/2 -> PwrInfo/1  "<PwrInfo>"
  Demux1/2 -> Bus Creator7/2  "WhlAngRR"
  Demux1/1 -> Bus Creator7/1  "WhlAngRL"
  Demux/2 -> Bus Creator8/2  "WhlAngFR"
  Demux/1 -> Bus Creator8/1  "WhlAngFL"
  Bus Creator8/1 -> Bus Creator5/3  "Steer"
  Bus Creator7/1 -> Bus Creator6/3  "Steer"
  WhlAngR/1 -> Demux1/1  "WhlAngR"
  WhlAngF/1 -> Demux/1  "WhlAngF"
  Hard Point Coordinate Transform Geometric/1(Inert) -> Bus Creator2/5  "Geom"
  Hard Point Coordinate Transform Geometric/2(Body) -> Bus Creator1/8  "Geom"
  Forces/1 -> Bus Creator1/2  "Forces"
  BdyFrmCg/1 -> Hard Point Coordinate Transform Front Left/2(BdyFrmCg), Hard Point Coordinate Transform Front Right/2(BdyFrmCg), Hard Point Coordinate Transform Rear Left/2(BdyFrmCg), Hard Point Coordinate Transform Rear Right/2(BdyFrmCg), Hitch Coordinate Transform/2(BodyFrmCg), Bus Creator1/1, Hard Point Coordinate Transform Geometric/2(BdyFrmCg)  "Cg"
  Bus Creator3/1 -> Bus Creator2/2  "FrntAxl"
  Bus Creator1/1 -> BdyFrm/1  "BdyFrm"
  Bus Creator2/1 -> InertFrm/1  "InertFrm"
  Bus Creator4/1 -> Bus Creator2/3  "RearAxl"
  InertCg/1 -> Hard Point Coordinate Transform Rear Left/1(InertFrmCg), Hard Point Coordinate Transform Rear Right/1(InertFrmCg), Hard Point Coordinate Transform Geometric/1(InertFrmCg), Hitch Coordinate Transform/1(InertFrmCg), Hard Point Coordinate Transform Front Right/1(InertFrmCg), Bus Creator2/1, Hard Point Coordinate Transform Front Left/1(InertFrmCg)  "Cg"
  Bus Creator5/1 -> Bus Creator1/4  "FrntAxl"
  Moments/1 -> Bus Creator1/3  "Moments"
  Hard Point Coordinate Transform Front Left/1(Inert) -> Bus Creator3/1  "Lft"
  Hard Point Coordinate Transform Front Right/1(Inert) -> Bus Creator3/2  "Rght"
  Hard Point Coordinate Transform Rear Left/1(Inert) -> Bus Creator4/1  "Lft"
  Hard Point Coordinate Transform Rear Right/1(Inert) -> Bus Creator4/2  "Rght"
  Hard Point Coordinate Transform Rear Right/2(Body) -> Bus Creator6/2  "Rght"
  Hard Point Coordinate Transform Rear Left/2(Body) -> Bus Creator6/1  "Lft"
  Hard Point Coordinate Transform Front Right/2(Body) -> Bus Creator5/2  "Rght"
  Hard Point Coordinate Transform Front Left/2(Body) -> Bus Creator5/1  "Lft"
  Bus Creator6/1 -> Bus Creator1/5  "RearAxl"

== system PassVeh7DOF/Vehicle Body 3DOF External Longitudinal Wheels/Dual/Vehicle Body 3DOF Dual Track/Signal Routing/Signal Routing Dual/Moments ==
  MBody : Inport
  Mdrag : Inport  Port=2
  MExt : Inport  Port=3
  Mh : Inport  Port=4
  Bus Creator{1..3,24} (4 alike) : BusCreator  Inputs=3
  Bus Creator7 : BusCreator  Inputs=4
  Demux{,1..3} (4 alike) : Demux  Outputs=3
  Signal Specification{1..11,23} (12 alike) : SignalSpecification  Unit=N*m
  Moments : Outport  VectorParamsAs1DForOutWhenUnconnected=off
  wires:
  Signal Specification11/1 -> Bus Creator2/1  "Mx"
  Demux3/1 -> Signal Specification11/1
  Demux3/3 -> Signal Specification10/1
  Bus Creator2/1 -> Bus Creator7/4  "Hitch"
  Demux3/2 -> Signal Specification9/1
  Signal Specification9/1 -> Bus Creator2/2  "My"
  Mh/1 -> Demux3/1
  Signal Specification10/1 -> Bus Creator2/3  "Mz"
  Signal Specification23/1 -> Bus Creator24/1  "Mx"
  Bus Creator24/1 -> Bus Creator7/1  "Body"
  Signal Specification1/1 -> Bus Creator24/2  "My"
  Signal Specification2/1 -> Bus Creator24/3  "Mz"
  Bus Creator1/1 -> Bus Creator7/2  "Drag"
  Bus Creator7/1 -> Moments/1  "Moments"
  Demux/2 -> Signal Specification1/1
  Demux/1 -> Signal Specification23/1
  Demux/3 -> Signal Specification2/1
  MBody/1 -> Demux/1
  Mdrag/1 -> Demux1/1
  Demux1/3 -> Signal Specification4/1
  Demux1/1 -> Signal Specification5/1
  Demux1/2 -> Signal Specification3/1
  Signal Specification4/1 -> Bus Creator1/3  "Mz"
  Signal Specification3/1 -> Bus Creator1/2  "My"
  Signal Specification5/1 -> Bus Creator1/1  "Mx"
  MExt/1 -> Demux2/1
  Signal Specification7/1 -> Bus Creator3/3  "Mz"
  Signal Specification6/1 -> Bus Creator3/2  "My"
  Bus Creator3/1 -> Bus Creator7/3  "Ext"
  Signal Specification8/1 -> Bus Creator3/1  "Mx"
  Demux2/2 -> Signal Specification6/1
  Demux2/1 -> Signal Specification8/1
  Demux2/3 -> Signal Specification7/1

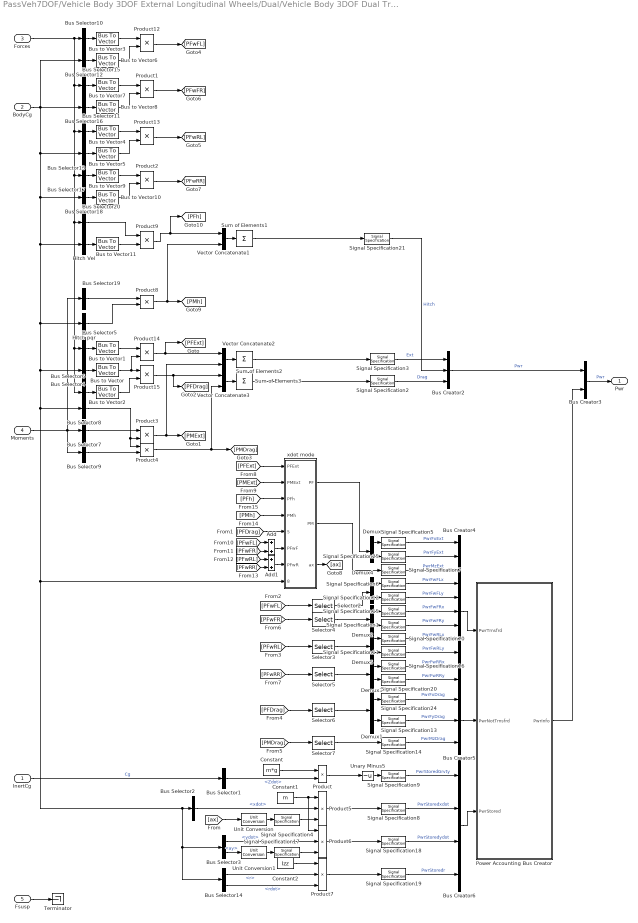
== system PassVeh7DOF/Vehicle Body 3DOF External Longitudinal Wheels/Dual/Vehicle Body 3DOF Dual Track/Signal Routing/Signal Routing Dual/Power ==
  InertCg : Inport
  BodyCg : Inport  Port=2
  Forces : Inport  Port=3
  Moments : Inport  Port=4
  Fsusp : Inport  Port=5
  Add : Sum
  Add1 : Sum
  Bus Creator2 : BusCreator  Inputs=3
  Bus Creator3 : BusCreator  Inputs=2
  Bus Creator4 : BusCreator  Inputs=11
  Bus Creator5 : BusCreator  Inputs=3
  Bus Creator6 : BusCreator  Inputs=4
  Bus Selector1 : BusSelector  OutputSignals=Cg.Vel.Zdot
  Bus Selector10 : BusSelector  OutputSignals=FrntAxl.Lft.Fx,FrntAxl.Lft.Fy,FrntAxl.Lft.Fz  OutputAsBus=on
  Bus Selector11 : BusSelector  OutputSignals=RearAxl.Lft.Fx,RearAxl.Lft.Fy,RearAxl.Lft.Fz  OutputAsBus=on
  Bus Selector12 : BusSelector  OutputSignals=FrntAxl.Lft.Vel.xdot,FrntAxl.Lft.Vel.ydot,FrntAxl.Lft.Vel.zdot  OutputAsBus=on
  Bus Selector13 : BusSelector  OutputSignals=RearAxl.Lft.Vel.xdot,RearAxl.Lft.Vel.ydot,RearAxl.Lft.Vel.zdot  OutputAsBus=on
  Bus Selector14 : BusSelector  OutputSignals=Cg.AngVel.r,Cg.AngAcc.rdot
  Bus Selector15 : BusSelector  OutputSignals=FrntAxl.Rght.Fx,FrntAxl.Rght.Fy,FrntAxl.Rght.Fz  OutputAsBus=on
  Bus Selector16 : BusSelector  OutputSignals=FrntAxl.Rght.Vel.xdot,FrntAxl.Rght.Vel.ydot,FrntAxl.Rght.Vel.zdot  OutputAsBus=on
  Bus Selector17 : BusSelector  OutputSignals=RearAxl.Rght.Fx,RearAxl.Rght.Fy,RearAxl.Rght.Fz  OutputAsBus=on
  Bus Selector18 : BusSelector  OutputSignals=RearAxl.Rght.Vel.xdot,RearAxl.Rght.Vel.ydot,RearAxl.Rght.Vel.zdot  OutputAsBus=on
  Bus Selector19 : BusSelector  OutputSignals=Hitch.Mx,Hitch.My,Hitch.Mz  OutputAsBus=on
  Bus Selector2 : BusSelector  OutputSignals=Cg.Vel.xdot
  Bus Selector20 : BusSelector  OutputSignals=Hitch.Fx,Hitch.Fy,Hitch.Fz  OutputAsBus=on
  Bus Selector3 : BusSelector  OutputSignals=Cg.Vel.ydot,Cg.Acc.ay
  Bus Selector4 : BusSelector  OutputSignals=Cg.Vel.xdot,Cg.Vel.ydot,Cg.Vel.zdot  OutputAsBus=on
  Bus Selector5 : BusSelector  OutputSignals=Ext.Fx,Ext.Fy,Ext.Fz  OutputAsBus=on
  Bus Selector6 : BusSelector  OutputSignals=Drag.Fx,Drag.Fy,Drag.Fz  OutputAsBus=on
  Bus Selector7 : BusSelector  OutputSignals=Ext.Mx,Ext.My,Ext.Mz  OutputAsBus=on
  Bus Selector8 : BusSelector  OutputSignals=Cg.AngVel.p,Cg.AngVel.q,Cg.AngVel.r  OutputAsBus=on
  Bus Selector9 : BusSelector  OutputSignals=Drag.Mx,Drag.My,Drag.Mz  OutputAsBus=on
  Bus to Vector{,1..11} (12 alike) : BusToVector
  Constant : Constant  Value=m*g
  Constant1 : Constant  Value=m
  Constant2 : Constant  Value=Izz
  Demux{,1..5} (6 alike) : Demux  Outputs=2
  Hitch Vel : BusSelector  OutputSignals=Hitch.Vel.xdot,Hitch.Vel.ydot,Hitch.Vel.zdot  OutputAsBus=on
  Hitch pqr : BusSelector  OutputSignals=Cg.AngVel.p,Cg.AngVel.q,Cg.AngVel.r  OutputAsBus=on
  Power Accounting Bus Creator : Subsystem  mask(Power Accounting Bus Creator){AssctBlkSelPopup=Parent reference block, RefBlkName='autolibshared/Vehicle Body 3DOF Single Track', PwrTrnsfrdCheckBox=on, PwrNotTrnsfrdCheckBox=on, PwrStoredCheckBox=on, aMode=aMode}
      mask prompts: AssctBlkSelPopup "autoblks_shared:autoblkPwrInfoBus:assocBlkSel"; RefBlkName "autoblks_shared:autoblkPwrInfoBus:refBlkName"
      mask init:
      | autosharedicon('autolibpowerbusutil', gcb, 'Initialization')
      settings: ModelCloseFcn=autosharedicon('autolibpowerbusutil', gcb, 'CloseFcn')  OpenFcn=autosharedicon('autolibpowerbusutil', gcb, 'OpenFcn')  CloseFcn=autosharedicon('autolibpowerbusutil', gcb, 'CloseFcn')
      mask Help: eval('autosharedhelp(''pbpwrbuscreator'')');
      mask TypeOptions AssctBlkSelPopup: Parent | Parent reference block
      mask DialogControl AssctBlkSelPopup Prompt: Associated block selection:
      mask DialogControl RefBlkName Prompt: Reference block name:
  Product{,1..4,8..9,12..15} (11 alike) : Product
  Product5 : Product  Inputs=3
  Product6 : Product  Inputs=3
  Product7 : Product  Inputs=3
  Selector{2..6} (5 alike) : Selector  InputPortWidth=3  IndexOptions=Index vector (dialog)  Indices=[1 2]  OutputSizes=1
  Selector7 : Selector  InputPortWidth=3  IndexOptions=Index vector (dialog)  Indices=[3]  OutputSizes=1
  Signal Specification{1..3,5..16,18..21,24..25} (21 alike) : SignalSpecification  Unit=W
  Signal Specification17 : SignalSpecification  Unit=m/s^2
  Signal Specification4 : SignalSpecification  Unit=m/s^2
  Sum of Elements1 : Sum  Inputs=+
  Sum of Elements2 : Sum  Inputs=+
  Sum of Elements3 : Sum  Inputs=+
  Terminator : Terminator
  Unary Minus5 : UnaryMinus
  Unit Conversion : UnitConversion
  Unit Conversion1 : UnitConversion
  Vector Concatenate1 : Concatenate
  Vector Concatenate2 : Concatenate
  Vector Concatenate3 : Concatenate
  xdot mode : Subsystem  Variant=on  VariantControlMode=label  LabelModeActiveChoice=1
  Pwr : Outport  VectorParamsAs1DForOutWhenUnconnected=off
  wires:
  [PMh] -> xdot mode/4(PMh)
  [PFh] -> xdot mode/3(PFh)
  Vector Concatenate1/1 -> Sum of Elements1/1
  Forces/1 -> Bus Selector10/1, Bus Selector11/1, Bus Selector5/1, Bus Selector6/1, Bus Selector20/1, Bus Selector17/1, Bus Selector15/1
  BodyCg/1 -> Bus Selector12/1, Bus Selector13/1, Bus Selector4/1, Bus Selector8/1, xdot mode/8(BodyFrm), Bus Selector3/1, Bus Selector14/1, Bus Selector2/1, Hitch pqr/1, Hitch Vel/1, Bus Selector18/1, Bus Selector16/1
  Signal Specification21/1 -> Bus Creator2/2  "Hitch"
  Hitch Vel/1 -> Bus to Vector11/1
  Bus to Vector11/1 -> Product9/2
  Product9/1 -> Vector Concatenate1/1, [PFh]
  Sum of Elements1/1 -> Signal Specification21/1
  Bus Selector20/1 -> Product9/1
  Hitch pqr/1 -> Product8/2
  Bus Selector19/1 -> Product8/1
  Product8/1 -> [PMh], Vector Concatenate1/2
  Signal Specification16/1 -> Bus Creator4/10  "PwrFwRRx"
  [PFwRR] -> Selector5/1
  Signal Specification20/1 -> Bus Creator4/11  "PwrFwRRy"
  Demux3/2 -> Signal Specification20/1
  Selector5/1 -> Demux3/1
  Demux3/1 -> Signal Specification16/1
  [PFwFR] -> Selector4/1
  Signal Specification15/1 -> Bus Creator4/6  "PwrFwFRx"
  Signal Specification1/1 -> Bus Creator4/7  "PwrFwFRy"
  Selector4/1 -> Demux2/1
  Demux2/1 -> Signal Specification15/1
  Demux2/2 -> Signal Specification1/1
  Bus Selector17/1 -> Bus to Vector9/1
  Product2/1 -> [PFwRR]
  Bus Selector18/1 -> Bus to Vector10/1
  Bus to Vector9/1 -> Product2/1
  Bus to Vector10/1 -> Product2/2
  Bus Selector16/1 -> Bus to Vector8/1
  Product1/1 -> [PFwFR]
  Bus Selector15/1 -> Bus to Vector7/1
  Bus to Vector8/1 -> Product1/2
  Bus to Vector7/1 -> Product1/1
  Fsusp/1 -> Terminator/1
  Product4/1 -> [PMDrag], Vector Concatenate3/2
  Power Accounting Bus Creator/1(PwrInfo) -> Bus Creator3/2
  Unit Conversion/1 -> Signal Specification4/1
  Demux4/2 -> Signal Specification12/1
  Constant/1 -> Product/1
  Product6/1 -> Signal Specification18/1
  Demux/1 -> Signal Specification5/1
  Bus to Vector5/1 -> Product13/2
  Product/1 -> Unary Minus5/1
  Signal Specification25/1 -> Bus Creator4/2  "PwrFyExt"
  Constant1/1 -> Product6/1, Product5/1
  Bus to Vector/1 -> Product14/2, Product15/1
  Signal Specification5/1 -> Bus Creator4/1  "PwrFxExt"
  Demux5/1 -> Signal Specification10/1
  Signal Specification24/1 -> Bus Creator5/1  "PwrFxDrag"
  Unary Minus5/1 -> Signal Specification9/1
  Product12/1 -> [PFwFL]
  Demux1/1 -> Signal Specification24/1
  Demux4/1 -> Signal Specification6/1
  Selector3/1 -> Demux5/1
  Bus Selector9/1 -> Product4/2
  Signal Specification17/1 -> Product6/3
  Demux5/2 -> Signal Specification11/1
  Selector2/1 -> Demux4/1
  Signal Specification12/1 -> Bus Creator4/5  "PwrFwFLy"
  Unit Conversion1/1 -> Signal Specification17/1
  Signal Specification10/1 -> Bus Creator4/8  "PwrFwRLx"
  Bus Selector8/1 -> Product3/2, Product4/1
  Signal Specification2/1 -> Bus Creator2/3  "Drag"
  Bus Selector7/1 -> Product3/1
  xdot mode/2(PM) -> Signal Specification7/1
  Signal Specification11/1 -> Bus Creator4/9  "PwrFwRLy"
  Signal Specification9/1 -> Bus Creator6/1  "PwrStoredGrvty"
  Bus to Vector4/1 -> Product13/1
  Bus Creator3/1 -> Pwr/1  "Pwr"
  Signal Specification6/1 -> Bus Creator4/4  "PwrFwFLx"
  Bus Selector12/1 -> Bus to Vector6/1
  Selector6/1 -> Demux1/1
  [PFDrag] -> Selector6/1
  Signal Specification13/1 -> Bus Creator5/2  "PwrFyDrag"
  Bus to Vector3/1 -> Product12/1
  Bus Selector4/1 -> Bus to Vector/1
  Signal Specification7/1 -> Bus Creator4/3  "PwrMzExt"
  [PFwFL] -> Selector2/1
  [ax] -> Unit Conversion/1
  Signal Specification14/1 -> Bus Creator5/3  "PwrMzDrag"
  Demux1/2 -> Signal Specification13/1
  [PMDrag] -> Selector7/1
  Bus to Vector6/1 -> Product12/2
  Bus Selector10/1 -> Bus to Vector3/1
  xdot mode/1(PF) -> Demux/1
  Bus Selector14/1 -> Product7/2  "<r>"
  Bus Selector14/2 -> Product7/3  "<rdot>"
  Signal Specification18/1 -> Bus Creator6/3  "PwrStoredydot"
  Bus Selector3/2 -> Unit Conversion1/1  "<ay>"
  Vector Concatenate3/1 -> Sum of Elements3/1
  Bus Selector2/1 -> Product5/2  "<xdot>"
  Signal Specification19/1 -> Bus Creator6/4  "PwrStoredr"
  Vector Concatenate2/1 -> Sum of Elements2/1
  Moments/1 -> Bus Selector9/1, Bus Selector19/1, Bus Selector7/1
  Bus Selector13/1 -> Bus to Vector5/1
  Bus to Vector2/1 -> Product15/2
  Sum of Elements2/1 -> Signal Specification3/1
  Constant2/1 -> Product7/1
  Bus Selector3/1 -> Product6/2  "<ydot>"
  Product7/1 -> Signal Specification19/1
  Product13/1 -> [PFwRL]
  Selector7/1 -> Signal Specification14/1
  Demux/2 -> Signal Specification25/1
  [PFwRL] -> Selector3/1
  Signal Specification8/1 -> Bus Creator6/2  "PwrStoredxdot"
  Bus Selector6/1 -> Bus to Vector2/1
  Bus to Vector1/1 -> Product14/1
  Sum of Elements3/1 -> Signal Specification2/1
  InertCg/1 -> Bus Selector1/1  "Cg"
  Bus Selector11/1 -> Bus to Vector4/1
  Product3/1 -> Vector Concatenate2/2, [PMExt]
  Bus Selector1/1 -> Product/2  "<Zdot>"
  Signal Specification4/1 -> Product5/3
  Bus Selector5/1 -> Bus to Vector1/1
  Product14/1 -> Vector Concatenate2/1, [PFExt]
  Bus Creator2/1 -> Bus Creator3/1  "Pwr"
  Product15/1 -> Vector Concatenate3/1, [PFDrag]
  Signal Specification3/1 -> Bus Creator2/1  "Ext"
  Add/1 -> xdot mode/6(PFwF)
  [PFDrag] -> xdot mode/5(PFDrag)
  [PFExt] -> xdot mode/1(PFExt)
  [PMExt] -> xdot mode/2(PMExt)
  [PFwFL] -> Add/1
  [PFwFR] -> Add/2
  [PFwRL] -> Add1/1
  [PFwRR] -> Add1/2
  Add1/1 -> xdot mode/7(PFwR)
  Bus Creator5/1 -> Power Accounting Bus Creator/2(PwrNotTrnsfrd)
  Bus Creator4/1 -> Power Accounting Bus Creator/1(PwrTrnsfrd)
  Bus Creator6/1 -> Power Accounting Bus Creator/3(PwrStored)
  Product5/1 -> Signal Specification8/1
  xdot mode/3(ax) -> [ax]
